simulink model "MATLAB Simulink Model"  (R2020b)
settings: Solver=ode4  StartTime=0.0  StopTime=1  RelTol=1e-3
InitFcn:
  | clear;
  | clc;
  | 
  | %Motor Parameters
  | r1 = 1.405;
  | l1  = 0.005839;
  | r2 = 1.395;
  | l2 = 0.005839;
  | Lm = 0.1722;
  | 
  | %Motor Rated Values
  | Vrat = 400;
  | frat = 50;
  | 
  | x1 = 2*pi*frat*l1;
  | x2 = 2*pi*frat*l2;
  | Xm = 2*pi*frat*Lm;
  | Prat = 4*1000;
  | Nrat = 1430;
  | Ns = 120*frat/4;
  | nrat = Nrat*2*pi/60;
  | ns = Ns*2*pi/60;
  | srat = (Ns-Nrat)/Ns;
  | 
  | E1 = Vrat/sqrt(3); %phase voltage
  | IL = E1/( (r1 + (1i*x1) ) + ( ( (1i*x2) +(r2/srat) )*1i*Xm / ( (1i*Xm) + (1i*x2) + (r2/srat) ) ) );
  | E2 = E1 - (IL*(r1 + (1i*x1) ) );
  | Trat = (3/(ns))*srat*abs(E2)*abs(E2)*r2/((r2*r2) + (srat*srat*x2*x2));
  | %Trat = Prat/nrat;
  | 
  | %System Variables
  | Tsys = (1e-6);
  | Ts = (100e-6);
  | freq = 50;
  | 
  | m=1*freq/50;
  | %m = 1 * (freq/50);
  | Vbus = (400*sqrt(2)*2/sqrt(3)) / (1.15);
  | 
  | Vref = (Vbus*sqrt(3)/2) * m;
  | delay = Ts/Tsys;
  | 
  | % Motor Starting Parameters
  | inc_time = 0.1;
  | 
  | %Motor Loading time
  | load_time = 0.5;
  | 
  | %No. of Hybrid Zones
  | numzones = 3;
  | 
  | %Load ML model Weights
  | 
  | W1R_s1 = readmatrix('Regression Weights\W1_subnet1_tmp_odd_90.xlsx');
  | b1R_s1 = readmatrix('Regression Weights\b1_subnet1_tmp_odd_90.xlsx');
  | W1R_s2 = readmatrix('Regression Weights\W1_subnet2_tmp_odd_90.xlsx');
  | b1R_s2 = readmatrix('Regression Weights\b1_subnet2_tmp_odd_90.xlsx');
  | 
  | W2R = readmatrix('Regression Weights\W2_subnet_tmp_odd_90.xlsx');
  | b2R = readmatrix('Regression Weights\b2_subnet_tmp_odd_90.xlsx');
  | ... (+9 lines)
libraries: powerlib x72, simulink x55, powerlib_meascontrol x15, dspstat3 x11, dspsigops x1
(part 2 of 5)

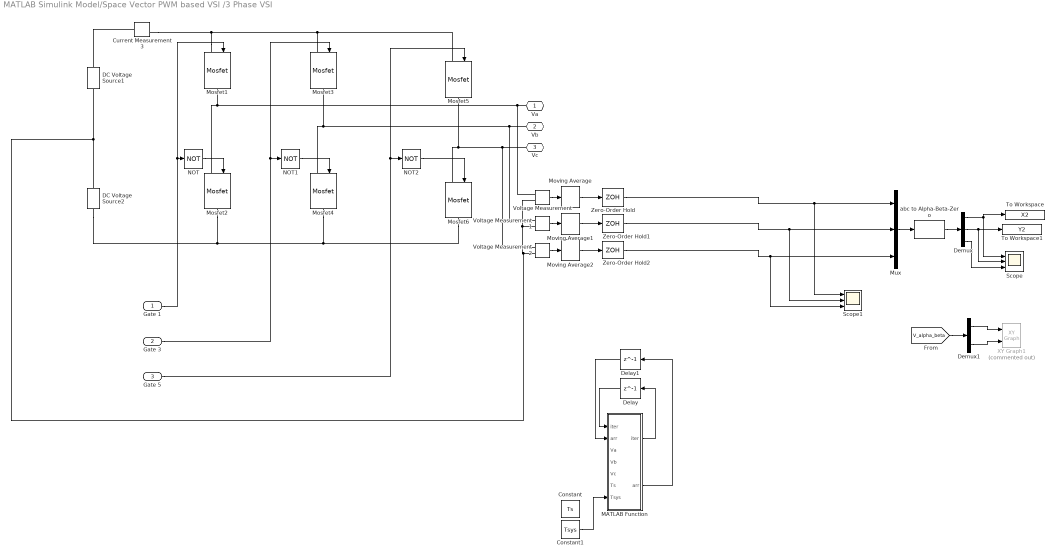
== system MATLAB Simulink Model/Space Vector PWM based VSI /3 Phase VSI ==
  Gate 1 : Inport
  Gate 3 : Inport  Port=2
  Gate 5 : Inport  Port=3
  Constant : Constant  Value=Ts  SampleTime=Tsys
  Constant1 : Constant  Value=Tsys  SampleTime=Tsys
  Current Measurement3 : powerlib/Measurements/Current Measurement  PhasorSimulation=off  OutputType=Complex  PSBequivalent=0
  DC Voltage Source1 : powerlib/Electrical Sources/DC Voltage Source  Amplitude=Vbus/2  Measurements=None
  DC Voltage Source2 : powerlib/Electrical Sources/DC Voltage Source  Amplitude=Vbus/2  Measurements=None
  Delay : Delay  DelayLength=1  SampleTime=Tsys
  Delay1 : Delay  DelayLength=1  SampleTime=Tsys
  Demux : Demux  Outputs=3
  Demux1 : Demux  Outputs=2
  MATLAB Function : MATLAB Function  TreatAsAtomicUnit=on
  Mosfet{1..6} (6 alike) : powerlib/Power Electronics/Mosfet  Ron=1e-6  Lon=0  Rd=1e-6  Vfd=0  IC=0  Rs=1e5  Cs=inf  Measurements=off
  Moving Average : dspstat3/Moving Average  Method=Sliding window  ForgettingFactorPort=off  SpecifyWindowLength=on  WindowLength=int8(Ts/Tsys)  ForgettingFactor=0.9  SimulateUsing=Code generation
  Moving Average1 : dspstat3/Moving Average  Method=Sliding window  ForgettingFactorPort=off  SpecifyWindowLength=on  WindowLength=int8(Ts/Tsys)  ForgettingFactor=0.9  SimulateUsing=Code generation
  Moving Average2 : dspstat3/Moving Average  Method=Sliding window  ForgettingFactorPort=off  SpecifyWindowLength=on  WindowLength=int8(Ts/Tsys)  ForgettingFactor=0.9  SimulateUsing=Code generation
  Mux : Mux  Inputs=3
  NOT : Logic  Operator=NOT  IconShape=distinctive  AllPortsSameDT=off  OutDataTypeStr=boolean
  NOT1 : Logic  Operator=NOT  IconShape=distinctive  AllPortsSameDT=off  OutDataTypeStr=boolean
  NOT2 : Logic  Operator=NOT  IconShape=distinctive  AllPortsSameDT=off  OutDataTypeStr=boolean
  Scope : Scope  NumInputPorts=3
  Scope1 : Scope  NumInputPorts=3
  To Workspace : ToWorkspace  VariableName=X2  SampleTime=-1
  To Workspace1 : ToWorkspace  VariableName=Y2  SampleTime=-1
  Voltage Measurement : powerlib/Measurements/Voltage Measurement  PhasorSimulation=off  OutputType=Complex  PSBequivalent=0
  Voltage Measurement1 : powerlib/Measurements/Voltage Measurement  PhasorSimulation=off  OutputType=Complex  PSBequivalent=0
  Voltage Measurement2 : powerlib/Measurements/Voltage Measurement  PhasorSimulation=off  OutputType=Complex  PSBequivalent=0
  XY Graph1 : simulink/Sinks/XY Graph  Commented=on  xmin=-Vref  xmax=Vref  ymin=-Vref  ymax=Vref  st=Ts
  Zero-Order Hold : ZeroOrderHold  SampleTime=Ts
  Zero-Order Hold1 : ZeroOrderHold  SampleTime=Ts
  Zero-Order Hold2 : ZeroOrderHold  SampleTime=Ts
  abc to Alpha-Beta-Zero : powerlib_meascontrol/Transformations/abc to Alpha-Beta-Zero
  Va : PMIOPort  Side=Right
  Vb : PMIOPort  Port=2  Side=Right
  Vc : PMIOPort  Port=3  Side=Right
  wires:
  Gate 3/1 -> NOT1/1, Mosfet3/1
  NOT1/1 -> Mosfet4/1
  Gate 1/1 -> NOT/1, Mosfet1/1
  Gate 5/1 -> NOT2/1, Mosfet5/1
  NOT/1 -> Mosfet2/1
  NOT2/1 -> Mosfet6/1
  Mux/1 -> abc to Alpha-Beta-Zero/1
  abc to Alpha-Beta-Zero/1 -> Demux/1
  Demux/1 -> To Workspace/1, Scope/1
  Demux/2 -> To Workspace1/1, Scope/2
  Demux/3 -> Scope/3
  [V_alpha_beta] -> Demux1/1
  Demux1/1 -> XY Graph1/1
  Demux1/2 -> XY Graph1/2
  Constant1/1 -> MATLAB Function/7(Tsys)
  MATLAB Function/1(iter) -> Delay/1
  Delay/1 -> MATLAB Function/1("iter ")
  Delay1/1 -> MATLAB Function/2("arr ")
  MATLAB Function/2(arr) -> Delay1/1
  Voltage Measurement/1 -> Moving Average/1
  Voltage Measurement1/1 -> Moving Average1/1
  Voltage Measurement2/1 -> Moving Average2/1
  Moving Average/1 -> Zero-Order Hold/1
  Moving Average1/1 -> Zero-Order Hold1/1
  Moving Average2/1 -> Zero-Order Hold2/1
  Zero-Order Hold/1 -> Scope1/1, Mux/1
  Zero-Order Hold1/1 -> Scope1/2, Mux/2
  Zero-Order Hold2/1 -> Scope1/3, Mux/3
  connections:
  Mosfet6/LConn1 -- Voltage Measurement2/LConn1 -- Vc/RConn1 -- Mosfet5/RConn1
  Mosfet4/LConn1 -- Voltage Measurement1/LConn1 -- Vb/RConn1 -- Mosfet3/RConn1
  Current Measurement3/LConn1 -- DC Voltage Source1/RConn1
  Mosfet1/LConn1 -- Current Measurement3/RConn1 -- Mosfet5/LConn1 -- Mosfet3/LConn1
  Mosfet2/LConn1 -- Voltage Measurement/LConn1 -- Va/RConn1 -- Mosfet1/RConn1
  Mosfet4/RConn1 -- DC Voltage Source2/LConn1 -- Mosfet2/RConn1 -- Mosfet6/RConn1
  DC Voltage Source2/RConn1 -- DC Voltage Source1/LConn1 -- Voltage Measurement1/LConn2 -- Voltage Measurement/LConn2 -- Voltage Measurement2/LConn2

== system MATLAB Simulink Model/Space Vector PWM based VSI /Gate Pulse Generator ==
  S1 : Inport
  S3 : Inport  Port=2
  S5 : Inport  Port=3
  sector : Inport  Port=4
  Constant : Constant  Value=Ts
  Constant1 : Constant  Value=Tsys
  Data Type Conversion : DataTypeConversion  OutDataTypeStr=boolean  RndMeth=Ceiling
  Data Type Conversion1 : DataTypeConversion  OutDataTypeStr=boolean  RndMeth=Ceiling
  Data Type Conversion2 : DataTypeConversion  OutDataTypeStr=boolean  RndMeth=Ceiling
  Delay : Delay  DelayLength=1
  Gate Pulse Values : MATLAB Function  TreatAsAtomicUnit=on
  Scope1 : Scope  NumInputPorts=5
  Gate 1 Pulse : Outport
  Gate 3 Pulse : Outport  Port=2
  Gate 5 Pulse : Outport  Port=3
  wires:
  sector/1 -> Scope1/5
  S1/1 -> Gate Pulse Values/2(S1)
  S3/1 -> Gate Pulse Values/3(S3)
  Gate Pulse Values/1(count) -> Delay/1
  Delay/1 -> Gate Pulse Values/1("count ")
  Gate Pulse Values/2(G1) -> Data Type Conversion/1
  Gate Pulse Values/3(G3) -> Data Type Conversion1/1
  Gate Pulse Values/4(G5) -> Data Type Conversion2/1
  Constant/1 -> Gate Pulse Values/5(Ts)
  Constant1/1 -> Gate Pulse Values/6(Tsys)
  S5/1 -> Gate Pulse Values/4(S5)
  Data Type Conversion/1 -> Gate 1 Pulse/1, Scope1/1
  Data Type Conversion1/1 -> Scope1/2, Gate 3 Pulse/1
  Data Type Conversion2/1 -> Gate 5 Pulse/1, Scope1/3
  [switchseq] -> Scope1/4

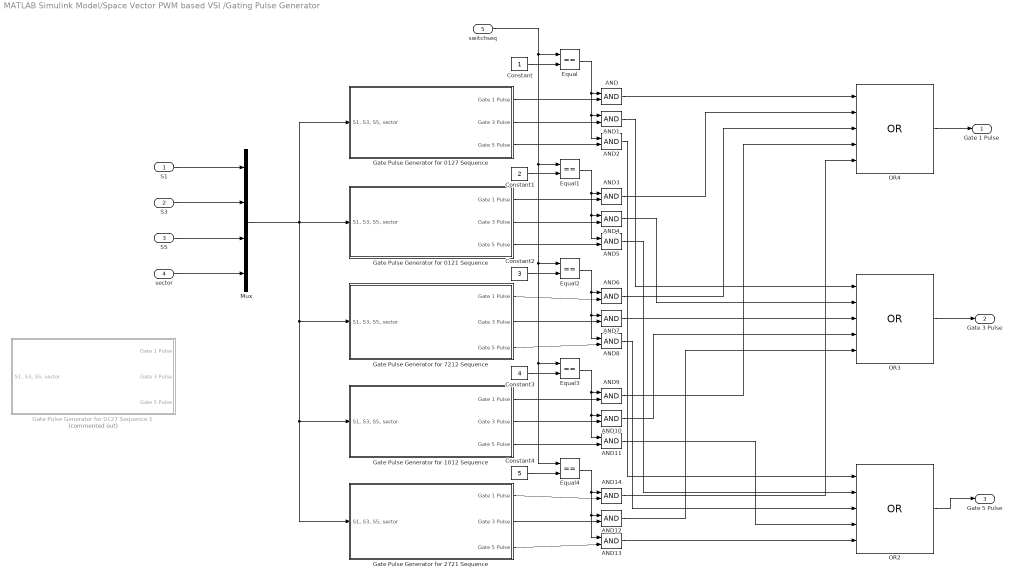
== system MATLAB Simulink Model/Space Vector PWM based VSI /Gating Pulse Generator ==
  S1 : Inport
  S3 : Inport  Port=2
  S5 : Inport  Port=3
  sector : Inport  Port=4
  switchseq : Inport  Port=5
  AND{,1..14} (15 alike) : Logic  IconShape=distinctive  AllPortsSameDT=off  OutDataTypeStr=boolean
  Constant : Constant
  Constant1 : Constant  Value=2
  Constant2 : Constant  Value=3
  Constant3 : Constant  Value=4
  Constant4 : Constant  Value=5
  Equal{,1..4} (5 alike) : RelationalOperator  Operator===  OutDataTypeStr=boolean  RndMeth=Simplest
  Gate Pulse Generator for 0121 Sequence : Subsystem
  Gate Pulse Generator for 0127 Sequence : Subsystem
  Gate Pulse Generator for 0127 Sequence 1 : Subsystem  Commented=on
  Gate Pulse Generator for 1012 Sequence : Subsystem
  Gate Pulse Generator for 2721 Sequence : Subsystem
  Gate Pulse Generator for 7212 Sequence : Subsystem
  Mux : Mux
  OR2 : Logic  Operator=OR  Inputs=5  IconShape=distinctive  AllPortsSameDT=off  OutDataTypeStr=boolean
  OR3 : Logic  Operator=OR  Inputs=5  IconShape=distinctive  AllPortsSameDT=off  OutDataTypeStr=boolean
  OR4 : Logic  Operator=OR  Inputs=5  IconShape=distinctive  AllPortsSameDT=off  OutDataTypeStr=boolean
  Gate 1 Pulse : Outport
  Gate 3 Pulse : Outport  Port=2
  Gate 5 Pulse : Outport  Port=3
  wires:
  sector/1 -> Mux/4
  S5/1 -> Mux/3
  S3/1 -> Mux/2
  S1/1 -> Mux/1
  Mux/1 -> Gate Pulse Generator for 0121 Sequence/1("S1, S3, S5, sector"), Gate Pulse Generator for 0127 Sequence/1("S1, S3, S5, sector"), Gate Pulse Generator for 7212 Sequence/1("S1, S3, S5, sector"), Gate Pulse Generator for 2721 Sequence/1("S1, S3, S5, sector"), Gate Pulse Generator for 1012 Sequence/1("S1, S3, S5, sector")
  Constant/1 -> Equal/2
  Equal/1 -> AND2/1, AND1/1, AND/1
  Gate Pulse Generator for 0121 Sequence/3(Gate 5 Pulse) -> AND5/2
  Gate Pulse Generator for 0121 Sequence/2(Gate 3 Pulse) -> AND4/2
  Equal1/1 -> AND3/1, AND4/1, AND5/1
  Gate Pulse Generator for 0121 Sequence/1(Gate 1 Pulse) -> AND3/2
  Constant1/1 -> Equal1/2
  Constant2/1 -> Equal2/2
  Gate Pulse Generator for 7212 Sequence/1(Gate 1 Pulse) -> AND6/2
  Equal2/1 -> AND8/1, AND7/1, AND6/1
  Gate Pulse Generator for 7212 Sequence/2(Gate 3 Pulse) -> AND7/2
  Gate Pulse Generator for 7212 Sequence/3(Gate 5 Pulse) -> AND8/2
  OR2/1 -> Gate 5 Pulse/1
  OR3/1 -> Gate 3 Pulse/1
  OR4/1 -> Gate 1 Pulse/1
  Gate Pulse Generator for 1012 Sequence/3(Gate 5 Pulse) -> AND11/2
  Gate Pulse Generator for 1012 Sequence/2(Gate 3 Pulse) -> AND10/2
  Equal3/1 -> AND10/1, AND11/1, AND9/1
  Gate Pulse Generator for 1012 Sequence/1(Gate 1 Pulse) -> AND9/2
  Constant3/1 -> Equal3/2
  switchseq/1 -> Equal/1, Equal4/1, Equal3/1, Equal2/1, Equal1/1
  Constant4/1 -> Equal4/2
  Gate Pulse Generator for 2721 Sequence/1(Gate 1 Pulse) -> AND14/2
  Equal4/1 -> AND14/1, AND13/1, AND12/1
  Gate Pulse Generator for 2721 Sequence/2(Gate 3 Pulse) -> AND12/2
  Gate Pulse Generator for 2721 Sequence/3(Gate 5 Pulse) -> AND13/2
  AND/1 -> OR4/1
  AND7/1 -> OR3/3
  AND13/1 -> OR2/5
  AND14/1 -> OR4/5
  AND3/1 -> OR4/2
  AND6/1 -> OR4/3
  AND9/1 -> OR4/4
  AND1/1 -> OR3/1
  AND4/1 -> OR3/2
  AND10/1 -> OR3/4
  AND12/1 -> OR3/5
  AND2/1 -> OR2/1
  AND5/1 -> OR2/2
  AND8/1 -> OR2/3
  AND11/1 -> OR2/4
  Gate Pulse Generator for 0127 Sequence/3(Gate 5 Pulse) -> AND2/2
  Gate Pulse Generator for 0127 Sequence/2(Gate 3 Pulse) -> AND1/2
  Gate Pulse Generator for 0127 Sequence/1(Gate 1 Pulse) -> AND/2

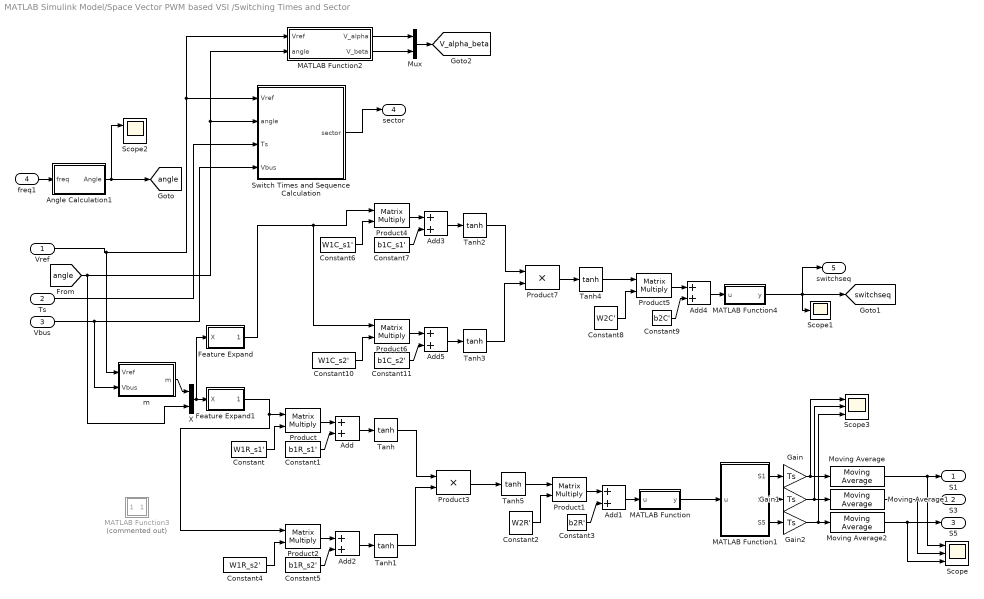
== system MATLAB Simulink Model/Space Vector PWM based VSI /Switching Times and Sector ==
  Vref : Inport
  Ts : Inport  Port=2
  Vbus : Inport  Port=3
  freq1 : Inport  Port=4
  Add{,1..5} (6 alike) : Sum
  Angle Calculation1 : Subsystem
  Constant : Constant  Value=W1R_s1'
  Constant1 : Constant  Value=b1R_s1'
  Constant10 : Constant  Value=W1C_s2'
  Constant11 : Constant  Value=b1C_s2'
  Constant2 : Constant  Value=W2R'
  Constant3 : Constant  Value=b2R'
  Constant4 : Constant  Value=W1R_s2'
  Constant5 : Constant  Value=b1R_s2'
  Constant6 : Constant  Value=W1C_s1'
  Constant7 : Constant  Value=b1C_s1'
  Constant8 : Constant  Value=W2C'
  Constant9 : Constant  Value=b2C'
  Feature Expand : MATLAB Function  TreatAsAtomicUnit=on
  Feature Expand1 : MATLAB Function  TreatAsAtomicUnit=on
  Gain : Gain  Gain=Ts
  Gain1 : Gain  Gain=Ts
  Gain2 : Gain  Gain=Ts
  MATLAB Function : MATLAB Function  TreatAsAtomicUnit=on
  MATLAB Function1 : MATLAB Function  TreatAsAtomicUnit=on
  MATLAB Function2 : MATLAB Function  TreatAsAtomicUnit=on
  MATLAB Function3 : MATLAB Function  Commented=on  TreatAsAtomicUnit=on
  MATLAB Function4 : MATLAB Function  TreatAsAtomicUnit=on
  Moving Average : dspstat3/Moving Average  Method=Sliding window  ForgettingFactorPort=off  SpecifyWindowLength=on  WindowLength=1  ForgettingFactor=0.9  SimulateUsing=Code generation
  Moving Average1 : dspstat3/Moving Average  Method=Sliding window  ForgettingFactorPort=off  SpecifyWindowLength=on  WindowLength=1  ForgettingFactor=0.9  SimulateUsing=Code generation
  Moving Average2 : dspstat3/Moving Average  Method=Sliding window  ForgettingFactorPort=off  SpecifyWindowLength=on  WindowLength=1  ForgettingFactor=0.9  SimulateUsing=Code generation
  Mux : Mux  Inputs=2
  Product{,1..2,4..6} (6 alike) : Product  Multiplication=Matrix(*)
  Product3 : Product
  Product7 : Product
  Scope : Scope  NumInputPorts=3
  Scope1 : Scope
  Scope2 : Scope  NumInputPorts=2
  Scope3 : Scope  NumInputPorts=3
  Switch Times and Sequence Calculation : MATLAB Function  TreatAsAtomicUnit=on
  Tanh{,1..5} (6 alike) : Trigonometry  Operator=tanh
  X : Concatenate
  m : MATLAB Function  TreatAsAtomicUnit=on
  S1 : Outport
  S3 : Outport  Port=2
  S5 : Outport  Port=3
  sector : Outport  Port=4
  switchseq : Outport  Port=5
  tag scope: V_alpha_beta=global, angle=global, switchseq=global
  wires:
  Vref/1 -> m/1(Vref), MATLAB Function2/1(Vref), Switch Times and Sequence Calculation/1(Vref)
  Ts/1 -> Switch Times and Sequence Calculation/3(Ts)
  [angle] -> X/2, MATLAB Function2/2(angle), Switch Times and Sequence Calculation/2(angle)
  Switch Times and Sequence Calculation/1(sector) -> sector/1
  Constant/1 -> Product/2
  Product/1 -> Add/1
  Constant1/1 -> Add/2
  Constant3/1 -> Add1/2
  Product1/1 -> Add1/1
  Constant2/1 -> Product1/2
  Add/1 -> Tanh/1
  Add1/1 -> MATLAB Function/1(u)
  MATLAB Function/1(y) -> MATLAB Function1/1(u)
  X/1 -> Feature Expand/1(X), Feature Expand1/1(X)
  freq1/1 -> Angle Calculation1/1(freq)
  Angle Calculation1/1(Angle) -> Scope2/1, [angle]
  MATLAB Function1/1(S1) -> Gain/1
  MATLAB Function1/3(S5) -> Gain2/1
  MATLAB Function1/2(S3) -> Gain1/1
  m/1(m) -> X/1
  Vbus/1 -> m/2(Vbus), Switch Times and Sequence Calculation/4(Vbus)
  Add2/1 -> Tanh1/1
  Constant5/1 -> Add2/2
  Product2/1 -> Add2/1
  Constant4/1 -> Product2/2
  Tanh1/1 -> Product3/2
  Tanh/1 -> Product3/1
  MATLAB Function2/1(V_alpha) -> Mux/1
  MATLAB Function2/2(V_beta) -> Mux/2
  Mux/1 -> [V_alpha_beta]
  Tanh2/1 -> Product7/1
  Tanh3/1 -> Product7/2
  Constant10/1 -> Product6/2
  Product6/1 -> Add5/1
  Constant11/1 -> Add5/2
  Add5/1 -> Tanh3/1
  Feature Expand/1(new_X) -> Product4/1, Product6/1
  MATLAB Function4/1(y) -> switchseq/1, Scope1/1, [switchseq]
  Add4/1 -> MATLAB Function4/1(u)
  Add3/1 -> Tanh2/1
  Constant8/1 -> Product5/2
  Product5/1 -> Add4/1
  Constant9/1 -> Add4/2
  Constant7/1 -> Add3/2
  Product4/1 -> Add3/1
  Constant6/1 -> Product4/2
  Product7/1 -> Tanh4/1
  Tanh4/1 -> Product5/1
  Tanh5/1 -> Product1/1
  Product3/1 -> Tanh5/1
  Feature Expand1/1(new_X) -> Product/1, Product2/1
  Gain/1 -> Scope3/1, Moving Average/1
  Moving Average/1 -> Scope/1, S1/1
  Gain1/1 -> Scope3/2, Moving Average1/1
  Gain2/1 -> Scope3/3, Moving Average2/1
  Moving Average1/1 -> Scope/2, S3/1
  Moving Average2/1 -> Scope/3, S5/1

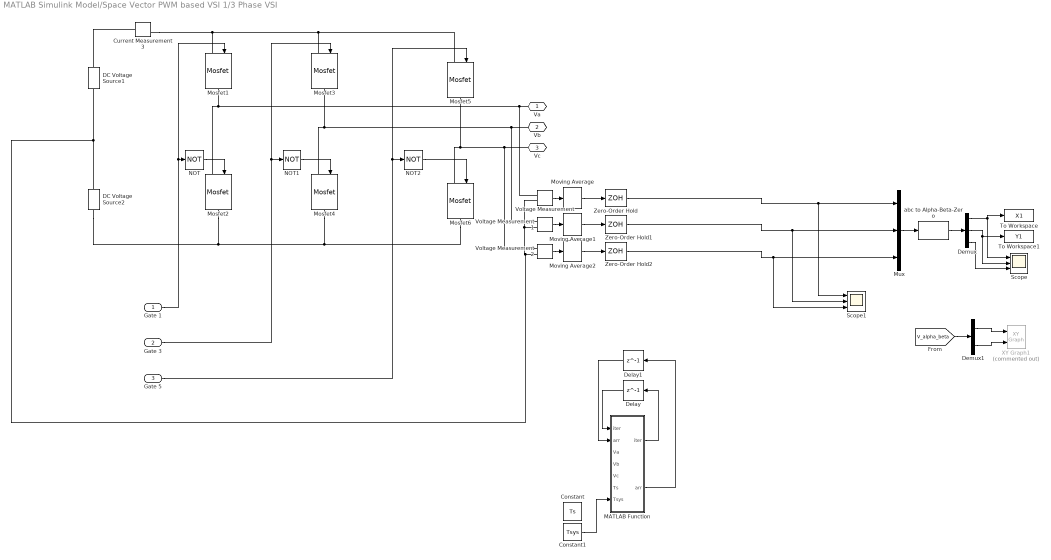
== system MATLAB Simulink Model/Space Vector PWM based VSI 1/3 Phase VSI ==
  Gate 1 : Inport
  Gate 3 : Inport  Port=2
  Gate 5 : Inport  Port=3
  Constant : Constant  Value=Ts  SampleTime=Tsys
  Constant1 : Constant  Value=Tsys  SampleTime=Tsys
  Current Measurement3 : powerlib/Measurements/Current Measurement  PhasorSimulation=off  OutputType=Complex  PSBequivalent=0
  DC Voltage Source1 : powerlib/Electrical Sources/DC Voltage Source  Amplitude=Vbus/2  Measurements=None
  DC Voltage Source2 : powerlib/Electrical Sources/DC Voltage Source  Amplitude=Vbus/2  Measurements=None
  Delay : Delay  DelayLength=1  SampleTime=Tsys
  Delay1 : Delay  DelayLength=1  SampleTime=Tsys
  Demux : Demux  Outputs=3
  Demux1 : Demux  Outputs=2
  MATLAB Function : MATLAB Function  TreatAsAtomicUnit=on
  Mosfet{1..6} (6 alike) : powerlib/Power Electronics/Mosfet  Ron=1e-6  Lon=0  Rd=1e-6  Vfd=0  IC=0  Rs=1e5  Cs=inf  Measurements=off
  Moving Average : dspstat3/Moving Average  Method=Sliding window  ForgettingFactorPort=off  SpecifyWindowLength=on  WindowLength=int8(Ts/Tsys)  ForgettingFactor=0.9  SimulateUsing=Code generation
  Moving Average1 : dspstat3/Moving Average  Method=Sliding window  ForgettingFactorPort=off  SpecifyWindowLength=on  WindowLength=int8(Ts/Tsys)  ForgettingFactor=0.9  SimulateUsing=Code generation
  Moving Average2 : dspstat3/Moving Average  Method=Sliding window  ForgettingFactorPort=off  SpecifyWindowLength=on  WindowLength=int8(Ts/Tsys)  ForgettingFactor=0.9  SimulateUsing=Code generation
  Mux : Mux  Inputs=3
  NOT : Logic  Operator=NOT  IconShape=distinctive  AllPortsSameDT=off  OutDataTypeStr=boolean
  NOT1 : Logic  Operator=NOT  IconShape=distinctive  AllPortsSameDT=off  OutDataTypeStr=boolean
  NOT2 : Logic  Operator=NOT  IconShape=distinctive  AllPortsSameDT=off  OutDataTypeStr=boolean
  Scope : Scope  NumInputPorts=3
  Scope1 : Scope  NumInputPorts=3
  To Workspace : ToWorkspace  VariableName=X1  SampleTime=-1
  To Workspace1 : ToWorkspace  VariableName=Y1  SampleTime=-1
  Voltage Measurement : powerlib/Measurements/Voltage Measurement  PhasorSimulation=off  OutputType=Complex  PSBequivalent=0
  Voltage Measurement1 : powerlib/Measurements/Voltage Measurement  PhasorSimulation=off  OutputType=Complex  PSBequivalent=0
  Voltage Measurement2 : powerlib/Measurements/Voltage Measurement  PhasorSimulation=off  OutputType=Complex  PSBequivalent=0
  XY Graph1 : simulink/Sinks/XY Graph  Commented=on  xmin=-Vref  xmax=Vref  ymin=-Vref  ymax=Vref  st=Ts
  Zero-Order Hold : ZeroOrderHold  SampleTime=Ts
  Zero-Order Hold1 : ZeroOrderHold  SampleTime=Ts
  Zero-Order Hold2 : ZeroOrderHold  SampleTime=Ts
  abc to Alpha-Beta-Zero : powerlib_meascontrol/Transformations/abc to Alpha-Beta-Zero
  Va : PMIOPort  Side=Right
  Vb : PMIOPort  Port=2  Side=Right
  Vc : PMIOPort  Port=3  Side=Right
  wires:
  Zero-Order Hold2/1 -> Mux/3, Scope1/3
  Zero-Order Hold1/1 -> Mux/2, Scope1/2
  Zero-Order Hold/1 -> Mux/1, Scope1/1
  Moving Average2/1 -> Zero-Order Hold2/1
  Moving Average1/1 -> Zero-Order Hold1/1
  Moving Average/1 -> Zero-Order Hold/1
  Voltage Measurement2/1 -> Moving Average2/1
  Voltage Measurement1/1 -> Moving Average1/1
  Voltage Measurement/1 -> Moving Average/1
  MATLAB Function/2(arr) -> Delay1/1
  Delay1/1 -> MATLAB Function/2("arr ")
  Delay/1 -> MATLAB Function/1("iter ")
  MATLAB Function/1(iter) -> Delay/1
  Constant1/1 -> MATLAB Function/7(Tsys)
  Demux1/2 -> XY Graph1/2
  Demux1/1 -> XY Graph1/1
  [V_alpha_beta] -> Demux1/1
  Demux/3 -> Scope/3
  Demux/2 -> To Workspace1/1, Scope/2
  Demux/1 -> To Workspace/1, Scope/1
  abc to Alpha-Beta-Zero/1 -> Demux/1
  Mux/1 -> abc to Alpha-Beta-Zero/1
  NOT2/1 -> Mosfet6/1
  NOT/1 -> Mosfet2/1
  Gate 5/1 -> Mosfet5/1, NOT2/1
  Gate 1/1 -> Mosfet1/1, NOT/1
  NOT1/1 -> Mosfet4/1
  Gate 3/1 -> Mosfet3/1, NOT1/1
  connections:
  Voltage Measurement2/LConn2 -- Voltage Measurement/LConn2 -- Voltage Measurement1/LConn2 -- DC Voltage Source1/LConn1 -- DC Voltage Source2/RConn1
  Mosfet6/RConn1 -- Mosfet2/RConn1 -- DC Voltage Source2/LConn1 -- Mosfet4/RConn1
  Mosfet1/RConn1 -- Va/RConn1 -- Voltage Measurement/LConn1 -- Mosfet2/LConn1
  Mosfet3/LConn1 -- Mosfet5/LConn1 -- Current Measurement3/RConn1 -- Mosfet1/LConn1
  Current Measurement3/LConn1 -- DC Voltage Source1/RConn1
  Mosfet3/RConn1 -- Vb/RConn1 -- Voltage Measurement1/LConn1 -- Mosfet4/LConn1
  Mosfet5/RConn1 -- Vc/RConn1 -- Voltage Measurement2/LConn1 -- Mosfet6/LConn1

== system MATLAB Simulink Model/Space Vector PWM based VSI 1/Gate Pulse Generator ==
  S1 : Inport
  S3 : Inport  Port=2
  S5 : Inport  Port=3
  sector : Inport  Port=4
  Constant : Constant  Value=Ts
  Constant1 : Constant  Value=Tsys
  Data Type Conversion : DataTypeConversion  OutDataTypeStr=boolean  RndMeth=Ceiling
  Data Type Conversion1 : DataTypeConversion  OutDataTypeStr=boolean  RndMeth=Ceiling
  Data Type Conversion2 : DataTypeConversion  OutDataTypeStr=boolean  RndMeth=Ceiling
  Delay : Delay  DelayLength=1
  Gate Pulse Values : MATLAB Function  TreatAsAtomicUnit=on
  Scope1 : Scope  NumInputPorts=5
  Gate 1 Pulse : Outport
  Gate 3 Pulse : Outport  Port=2
  Gate 5 Pulse : Outport  Port=3
  wires:
  [switchseq] -> Scope1/4
  Data Type Conversion2/1 -> Scope1/3, Gate 5 Pulse/1
  Data Type Conversion1/1 -> Gate 3 Pulse/1, Scope1/2
  Data Type Conversion/1 -> Scope1/1, Gate 1 Pulse/1
  S5/1 -> Gate Pulse Values/4(S5)
  Constant1/1 -> Gate Pulse Values/6(Tsys)
  Constant/1 -> Gate Pulse Values/5(Ts)
  Gate Pulse Values/4(G5) -> Data Type Conversion2/1
  Gate Pulse Values/3(G3) -> Data Type Conversion1/1
  Gate Pulse Values/2(G1) -> Data Type Conversion/1
  Delay/1 -> Gate Pulse Values/1("count ")
  Gate Pulse Values/1(count) -> Delay/1
  S3/1 -> Gate Pulse Values/3(S3)
  S1/1 -> Gate Pulse Values/2(S1)
  sector/1 -> Scope1/5

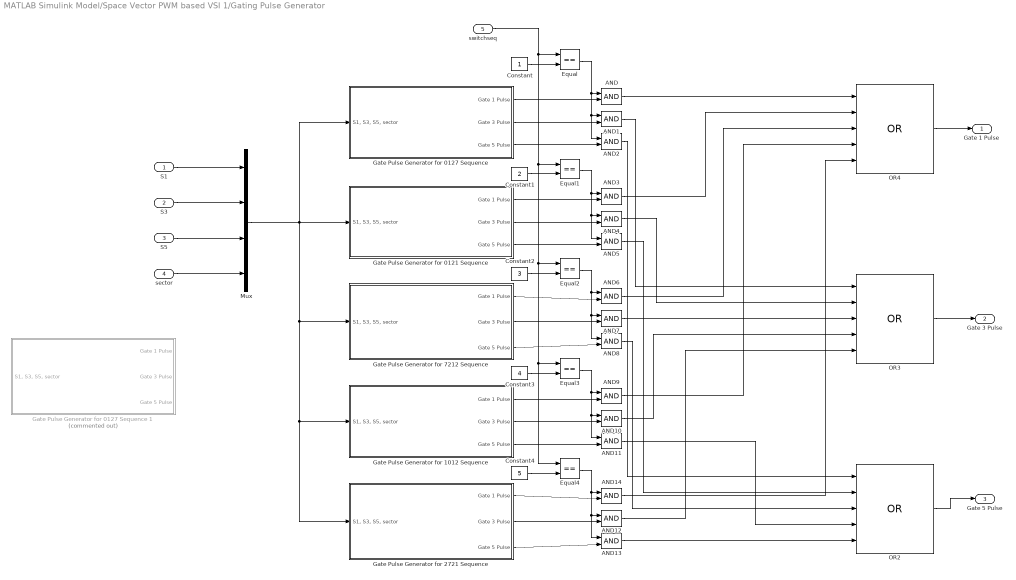
== system MATLAB Simulink Model/Space Vector PWM based VSI 1/Gating Pulse Generator ==
  S1 : Inport
  S3 : Inport  Port=2
  S5 : Inport  Port=3
  sector : Inport  Port=4
  switchseq : Inport  Port=5
  AND{,1..14} (15 alike) : Logic  IconShape=distinctive  AllPortsSameDT=off  OutDataTypeStr=boolean
  Constant : Constant
  Constant1 : Constant  Value=2
  Constant2 : Constant  Value=3
  Constant3 : Constant  Value=4
  Constant4 : Constant  Value=5
  Equal{,1..4} (5 alike) : RelationalOperator  Operator===  OutDataTypeStr=boolean  RndMeth=Simplest
  Gate Pulse Generator for 0121 Sequence : Subsystem
  Gate Pulse Generator for 0127 Sequence : Subsystem
  Gate Pulse Generator for 0127 Sequence 1 : Subsystem  Commented=on
  Gate Pulse Generator for 1012 Sequence : Subsystem
  Gate Pulse Generator for 2721 Sequence : Subsystem
  Gate Pulse Generator for 7212 Sequence : Subsystem
  Mux : Mux
  OR2 : Logic  Operator=OR  Inputs=5  IconShape=distinctive  AllPortsSameDT=off  OutDataTypeStr=boolean
  OR3 : Logic  Operator=OR  Inputs=5  IconShape=distinctive  AllPortsSameDT=off  OutDataTypeStr=boolean
  OR4 : Logic  Operator=OR  Inputs=5  IconShape=distinctive  AllPortsSameDT=off  OutDataTypeStr=boolean
  Gate 1 Pulse : Outport
  Gate 3 Pulse : Outport  Port=2
  Gate 5 Pulse : Outport  Port=3
  wires:
  Gate Pulse Generator for 0127 Sequence/1(Gate 1 Pulse) -> AND/2
  Gate Pulse Generator for 0127 Sequence/2(Gate 3 Pulse) -> AND1/2
  Gate Pulse Generator for 0127 Sequence/3(Gate 5 Pulse) -> AND2/2
  AND11/1 -> OR2/4
  AND8/1 -> OR2/3
  AND5/1 -> OR2/2
  AND2/1 -> OR2/1
  AND12/1 -> OR3/5
  AND10/1 -> OR3/4
  AND4/1 -> OR3/2
  AND1/1 -> OR3/1
  AND9/1 -> OR4/4
  AND6/1 -> OR4/3
  AND3/1 -> OR4/2
  AND14/1 -> OR4/5
  AND13/1 -> OR2/5
  AND7/1 -> OR3/3
  AND/1 -> OR4/1
  Gate Pulse Generator for 2721 Sequence/3(Gate 5 Pulse) -> AND13/2
  Gate Pulse Generator for 2721 Sequence/2(Gate 3 Pulse) -> AND12/2
  Equal4/1 -> AND12/1, AND13/1, AND14/1
  Gate Pulse Generator for 2721 Sequence/1(Gate 1 Pulse) -> AND14/2
  Constant4/1 -> Equal4/2
  switchseq/1 -> Equal1/1, Equal2/1, Equal3/1, Equal4/1, Equal/1
  Constant3/1 -> Equal3/2
  Gate Pulse Generator for 1012 Sequence/1(Gate 1 Pulse) -> AND9/2
  Equal3/1 -> AND9/1, AND11/1, AND10/1
  Gate Pulse Generator for 1012 Sequence/2(Gate 3 Pulse) -> AND10/2
  Gate Pulse Generator for 1012 Sequence/3(Gate 5 Pulse) -> AND11/2
  OR4/1 -> Gate 1 Pulse/1
  OR3/1 -> Gate 3 Pulse/1
  OR2/1 -> Gate 5 Pulse/1
  Gate Pulse Generator for 7212 Sequence/3(Gate 5 Pulse) -> AND8/2
  Gate Pulse Generator for 7212 Sequence/2(Gate 3 Pulse) -> AND7/2
  Equal2/1 -> AND6/1, AND7/1, AND8/1
  Gate Pulse Generator for 7212 Sequence/1(Gate 1 Pulse) -> AND6/2
  Constant2/1 -> Equal2/2
  Constant1/1 -> Equal1/2
  Gate Pulse Generator for 0121 Sequence/1(Gate 1 Pulse) -> AND3/2
  Equal1/1 -> AND5/1, AND4/1, AND3/1
  Gate Pulse Generator for 0121 Sequence/2(Gate 3 Pulse) -> AND4/2
  Gate Pulse Generator for 0121 Sequence/3(Gate 5 Pulse) -> AND5/2
  Equal/1 -> AND/1, AND1/1, AND2/1
  Constant/1 -> Equal/2
  Mux/1 -> Gate Pulse Generator for 1012 Sequence/1("S1, S3, S5, sector"), Gate Pulse Generator for 2721 Sequence/1("S1, S3, S5, sector"), Gate Pulse Generator for 7212 Sequence/1("S1, S3, S5, sector"), Gate Pulse Generator for 0127 Sequence/1("S1, S3, S5, sector"), Gate Pulse Generator for 0121 Sequence/1("S1, S3, S5, sector")
  S1/1 -> Mux/1
  S3/1 -> Mux/2
  S5/1 -> Mux/3
  sector/1 -> Mux/4

== system MATLAB Simulink Model/Space Vector PWM based VSI 1/Switching Times and Sector ==
  Vref : Inport
  Ts : Inport  Port=2
  Vbus : Inport  Port=3
  freq1 : Inport  Port=4
  Angle Calculation1 : Subsystem
  Scope : Scope  NumInputPorts=3
  Scope2 : Scope  NumInputPorts=2
  Switch Times and Sequence Calculation : MATLAB Function  TreatAsAtomicUnit=on
  S1 : Outport
  S3 : Outport  Port=2
  S5 : Outport  Port=3
  sector : Outport  Port=4
  switchseq : Outport  Port=5
  wires:
  ? -> ?
  Vbus/1 -> Switch Times and Sequence Calculation/4(Vbus)
  Angle Calculation1/1(Angle) -> Scope2/1
  freq1/1 -> Angle Calculation1/1(freq)
  Switch Times and Sequence Calculation/4(sector) -> sector/1
  [angle] -> Switch Times and Sequence Calculation/2(angle)
  Ts/1 -> Switch Times and Sequence Calculation/3(Ts)
  Vref/1 -> Switch Times and Sequence Calculation/1(Vref)
  Switch Times and Sequence Calculation/3(S5) -> Scope/3, S5/1
  Switch Times and Sequence Calculation/2(S3) -> Scope/2, S3/1
  Switch Times and Sequence Calculation/1(S1) -> Scope/1, S1/1
  Switch Times and Sequence Calculation/5(swseq) -> switchseq/1

== system MATLAB Simulink Model/15 Hz System/Space Vector PWM based VSI 1/3 Phase VSI ==
  Gate 1 : Inport
  Gate 3 : Inport  Port=2
  Gate 5 : Inport  Port=3
  Current Measurement3 : powerlib/Measurements/Current Measurement  PhasorSimulation=off  OutputType=Complex  PSBequivalent=0
  DC Voltage Source1 : powerlib/Electrical Sources/DC Voltage Source  Amplitude=Vbus  Measurements=None
  Mosfet{1..6} (6 alike) : powerlib/Power Electronics/Mosfet  Ron=1e-6  Lon=0  Rd=1e-6  Vfd=0  IC=0  Rs=1e5  Cs=inf  Measurements=on
  NOT : Logic  Operator=NOT  IconShape=distinctive  AllPortsSameDT=off  OutDataTypeStr=boolean
  NOT1 : Logic  Operator=NOT  IconShape=distinctive  AllPortsSameDT=off  OutDataTypeStr=boolean
  NOT2 : Logic  Operator=NOT  IconShape=distinctive  AllPortsSameDT=off  OutDataTypeStr=boolean
  Va : PMIOPort  Side=Right
  Vb : PMIOPort  Port=2  Side=Right
  Vc : PMIOPort  Port=3  Side=Right
  wires:
  Gate 3/1 -> NOT1/1, Mosfet3/1
  NOT1/1 -> Mosfet4/1
  Gate 1/1 -> NOT/1, Mosfet1/1
  Gate 5/1 -> NOT2/1, Mosfet5/1
  NOT/1 -> Mosfet2/1
  NOT2/1 -> Mosfet6/1
  connections:
  Mosfet6/LConn1 -- Vc/RConn1 -- Mosfet5/RConn1
  Mosfet4/LConn1 -- Vb/RConn1 -- Mosfet3/RConn1
  Current Measurement3/LConn1 -- DC Voltage Source1/RConn1
  Mosfet1/LConn1 -- Current Measurement3/RConn1 -- Mosfet5/LConn1 -- Mosfet3/LConn1
  Mosfet2/LConn1 -- Va/RConn1 -- Mosfet1/RConn1
  Mosfet4/RConn1 -- DC Voltage Source1/LConn1 -- Mosfet2/RConn1 -- Mosfet6/RConn1

== system MATLAB Simulink Model/15 Hz System/Space Vector PWM based VSI 1/Gate Pulse Generator ==
  "S1, S3, S5, sector" : Inport
  Carrier : simulink/Sources/Repeating Sequence  rep_seq_t=[0 Ts/2 Ts]  rep_seq_y=[Ts 0 Ts]
  Demux : Demux
  G1 : RelationalOperator  OutDataTypeStr=boolean  RndMeth=Simplest
  G3 : RelationalOperator  OutDataTypeStr=boolean  RndMeth=Simplest
  G5 : RelationalOperator  OutDataTypeStr=boolean  RndMeth=Simplest
  Scope : Scope  NumInputPorts=4
  Gate 1 Pulse : Outport
  Gate 3 Pulse : Outport  Port=2
  Gate 5 Pulse : Outport  Port=3
  tag scope: sector1=global
  wires:
  "S1, S3, S5, sector"/1 -> Demux/1
  Demux/4 -> [sector1], Scope/4
  Demux/2 -> G3/1
  Demux/1 -> G1/1
  Carrier/1 -> G5/2, G3/2, G1/2
  G1/1 -> Scope/1, Gate 1 Pulse/1
  Demux/3 -> G5/1
  G3/1 -> Scope/2, Gate 3 Pulse/1
  G5/1 -> Scope/3, Gate 5 Pulse/1

== system MATLAB Simulink Model/15 Hz System/Space Vector PWM based VSI 1/Switching Times and Sector ==
  Vref : Inport
  Ts : Inport  Port=2
  Vbus : Inport  Port=3
  Angle to Sector and Theta : Subsystem
  Mux3 : Mux
  PLL : powerlib_meascontrol/PLL/PLL  Fmin=45  Par_Init=[0, 50]  ParK=[180, 3200, 1]  TcD=1e-4  MaxRateChangeFreq=12  FilterCutOffFreq=25  Ts=0  AGC=on
      settings: SourceProductBaseCode=PS
  Scope : Scope
  Scope2 : Scope  NumInputPorts=2
  Scope3 : Scope  NumInputPorts=3
  Switching times of all switches : MATLAB Function  TreatAsAtomicUnit=on
  Vas : Sin  Frequency=2*pi*15  SampleTime=0
  "S1, S3, S5, sector" : Outport
  tag scope: wt1=global
  wires:
  Angle to Sector and Theta/1(Sector) -> Mux3/4, Switching times of all switches/4(sector)
  Angle to Sector and Theta/2(theta) -> Scope2/2, Switching times of all switches/2(theta)
  Switching times of all switches/2(S3) -> Scope3/2, Mux3/2
  Switching times of all switches/3(S5) -> Scope3/3, Mux3/3
  Ts/1 -> Switching times of all switches/3(Ts)
  PLL/2 -> [wt1], Angle to Sector and Theta/1(angle), Scope2/1
  Vas/1 -> PLL/1
  Switching times of all switches/1(S1) -> Scope3/1, Mux3/1
  PLL/1 -> Scope/1
  Mux3/1 -> "S1, S3, S5, sector"/1
  Vref/1 -> Switching times of all switches/1(Vref)
  Vbus/1 -> Switching times of all switches/5(Vbus)

== system MATLAB Simulink Model/Space Vector PWM based VSI /Gating Pulse Generator/Gate Pulse Generator for 0121 Sequence ==
  "S1, S3, S5, sector" : Inport
  AND{,1..5} (6 alike) : Logic  IconShape=distinctive  AllPortsSameDT=off  OutDataTypeStr=boolean
  Constant : Constant  Value=2
  Data Type Conversion : DataTypeConversion
  Demux : Demux
  For Even Sector : Subsystem
  For Odd Sector : Subsystem
  Mod : Math  Operator=mod  SaturateOnIntegerOverflow=on
  Mux : Mux  Inputs=3
  NOT : Logic  Operator=NOT  IconShape=distinctive  AllPortsSameDT=off  OutDataTypeStr=boolean
  OR : Logic  Operator=OR  IconShape=distinctive  AllPortsSameDT=off  OutDataTypeStr=boolean
  OR1 : Logic  Operator=OR  IconShape=distinctive  AllPortsSameDT=off  OutDataTypeStr=boolean
  OR2 : Logic  Operator=OR  IconShape=distinctive  AllPortsSameDT=off  OutDataTypeStr=boolean
  Scope1 : Scope  NumInputPorts=4
  Gate 1 Pulse : Outport
  Gate 3 Pulse : Outport  Port=2
  Gate 5 Pulse : Outport  Port=3
  wires:
  For Odd Sector/3(Gate 5 Pulse) -> AND5/1
  OR2/1 -> Scope1/3, Gate 5 Pulse/1
  OR1/1 -> Scope1/2, Gate 3 Pulse/1
  Demux/3 -> Mux/3
  AND4/1 -> OR1/1
  OR/1 -> Scope1/1, Gate 1 Pulse/1
  For Odd Sector/1(Gate 1 Pulse) -> AND3/1
  AND5/1 -> OR2/1
  Demux/2 -> Mux/2
  AND1/1 -> OR1/2
  AND/1 -> OR/2
  Demux/4 -> Scope1/4, Mod/1
  For Even Sector/3(Gate 5 Pulse) -> AND2/1
  For Odd Sector/2(Gate 3 Pulse) -> AND4/1
  For Even Sector/1(Gate 1 Pulse) -> AND/1
  Data Type Conversion/1 -> AND3/2, AND4/2, AND5/2, NOT/1
  AND2/1 -> OR2/2
  Demux/1 -> Mux/1
  Mux/1 -> For Even Sector/1("S1, S3, S5"), For Odd Sector/1("S1, S3, S5")
  For Even Sector/2(Gate 3 Pulse) -> AND1/1
  Constant/1 -> Mod/2
  NOT/1 -> AND/2, AND1/2, AND2/2
  Mod/1 -> Data Type Conversion/1
  "S1, S3, S5, sector"/1 -> Demux/1
  AND3/1 -> OR/1

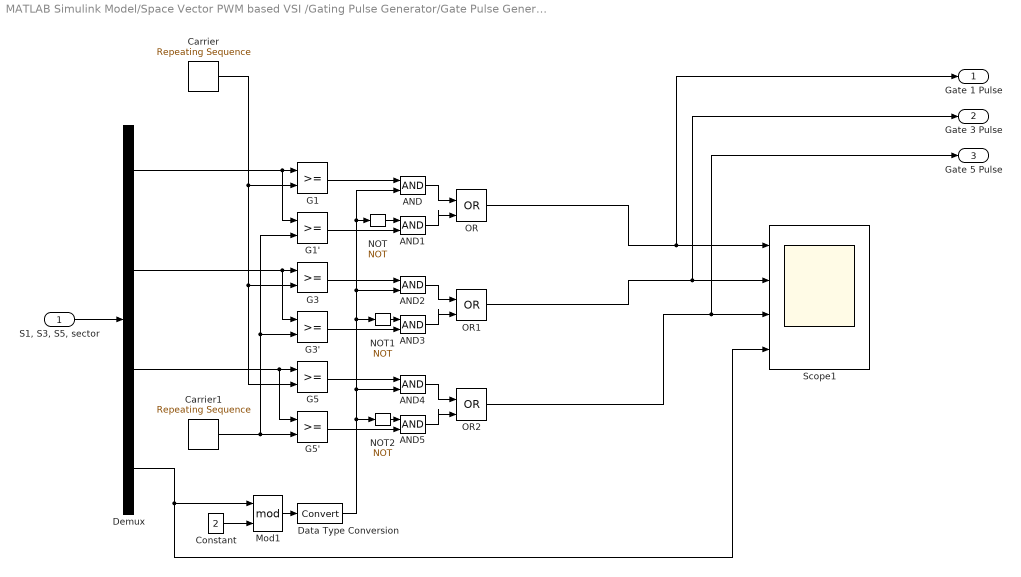
== system MATLAB Simulink Model/Space Vector PWM based VSI /Gating Pulse Generator/Gate Pulse Generator for 0127 Sequence ==
  "S1, S3, S5, sector" : Inport
  AND{,1..5} (6 alike) : Logic  IconShape=distinctive  AllPortsSameDT=off  OutDataTypeStr=boolean
  Carrier : simulink/Sources/Repeating Sequence  rep_seq_t=[0 Ts/2 Ts]  rep_seq_y=[Ts-(1e-16) 0 Ts-(1e-16)]
  Carrier1 : simulink/Sources/Repeating Sequence  rep_seq_t=[0 Ts/2 Ts]  rep_seq_y=[0 Ts-(1e-16) 0]
  Constant : Constant  Value=2
  Data Type Conversion : DataTypeConversion
  Demux : Demux
  G1 : RelationalOperator  OutDataTypeStr=boolean  RndMeth=Simplest
  G1' : RelationalOperator  OutDataTypeStr=boolean  RndMeth=Simplest
  G3 : RelationalOperator  OutDataTypeStr=boolean  RndMeth=Simplest
  G3' : RelationalOperator  OutDataTypeStr=boolean  RndMeth=Simplest
  G5 : RelationalOperator  OutDataTypeStr=boolean  RndMeth=Simplest
  G5' : RelationalOperator  OutDataTypeStr=boolean  RndMeth=Simplest
  Mod1 : Math  Operator=mod  SaturateOnIntegerOverflow=on
  NOT : Logic  Operator=NOT  IconShape=distinctive  AllPortsSameDT=off  OutDataTypeStr=boolean
  NOT1 : Logic  Operator=NOT  IconShape=distinctive  AllPortsSameDT=off  OutDataTypeStr=boolean
  NOT2 : Logic  Operator=NOT  IconShape=distinctive  AllPortsSameDT=off  OutDataTypeStr=boolean
  OR : Logic  Operator=OR  IconShape=distinctive  AllPortsSameDT=off  OutDataTypeStr=boolean
  OR1 : Logic  Operator=OR  IconShape=distinctive  AllPortsSameDT=off  OutDataTypeStr=boolean
  OR2 : Logic  Operator=OR  IconShape=distinctive  AllPortsSameDT=off  OutDataTypeStr=boolean
  Scope1 : Scope  NumInputPorts=4
  Gate 1 Pulse : Outport
  Gate 3 Pulse : Outport  Port=2
  Gate 5 Pulse : Outport  Port=3
  wires:
  G3/1 -> AND2/1
  OR2/1 -> Gate 5 Pulse/1, Scope1/3
  G3'/1 -> AND3/2
  OR/1 -> Gate 1 Pulse/1, Scope1/1
  Constant/1 -> Mod1/2
  AND1/1 -> OR/2
  Data Type Conversion/1 -> NOT2/1, AND4/2, NOT1/1, AND2/2, NOT/1, AND/2
  G5'/1 -> AND5/2
  G5/1 -> AND4/1
  AND5/1 -> OR2/2
  AND4/1 -> OR2/1
  AND/1 -> OR/1
  OR1/1 -> Scope1/2, Gate 3 Pulse/1
  NOT/1 -> AND1/1
  Mod1/1 -> Data Type Conversion/1
  AND3/1 -> OR1/2
  NOT2/1 -> AND5/1
  NOT1/1 -> AND3/1
  Carrier1/1 -> G1'/2, G3'/2, G5'/2
  Demux/1 -> G1'/1, G1/1
  G1'/1 -> AND1/2
  G1/1 -> AND/1
  Carrier/1 -> G5/2, G3/2, G1/2
  AND2/1 -> OR1/1
  "S1, S3, S5, sector"/1 -> Demux/1
  Demux/4 -> Scope1/4, Mod1/1
  Demux/2 -> G3'/1, G3/1
  Demux/3 -> G5'/1, G5/1

== system MATLAB Simulink Model/Space Vector PWM based VSI /Gating Pulse Generator/Gate Pulse Generator for 0127 Sequence 1 ==
  "S1, S3, S5, sector" : Inport
  AND{,1..5} (6 alike) : Logic  IconShape=distinctive  AllPortsSameDT=off  OutDataTypeStr=boolean
  Constant : Constant  Value=2
  Data Type Conversion : DataTypeConversion
  Demux : Demux
  For Even Sector : Subsystem
  For Odd Sector : Subsystem
  Mod : Math  Operator=mod  SaturateOnIntegerOverflow=on
  Mux : Mux  Inputs=3
  NOT : Logic  Operator=NOT  IconShape=distinctive  AllPortsSameDT=off  OutDataTypeStr=boolean
  OR : Logic  Operator=OR  IconShape=distinctive  AllPortsSameDT=off  OutDataTypeStr=boolean
  OR1 : Logic  Operator=OR  IconShape=distinctive  AllPortsSameDT=off  OutDataTypeStr=boolean
  OR2 : Logic  Operator=OR  IconShape=distinctive  AllPortsSameDT=off  OutDataTypeStr=boolean
  Scope1 : Scope  NumInputPorts=4
  Gate 1 Pulse : Outport
  Gate 3 Pulse : Outport  Port=2
  Gate 5 Pulse : Outport  Port=3
  wires:
  "S1, S3, S5, sector"/1 -> Demux/1
  Demux/1 -> Mux/1
  Demux/2 -> Mux/2
  Demux/3 -> Mux/3
  Mux/1 -> For Even Sector/1("S1, S3, S5"), For Odd Sector/1("S1, S3, S1")
  Demux/4 -> Scope1/4, Mod/1
  Constant/1 -> Mod/2
  Mod/1 -> Data Type Conversion/1
  NOT/1 -> AND/2, AND1/2, AND2/2
  For Odd Sector/1(Gate 1 Pulse1) -> AND3/1
  Data Type Conversion/1 -> AND3/2, AND4/2, AND5/2, NOT/1
  AND3/1 -> OR/1
  AND/1 -> OR/2
  AND4/1 -> OR1/1
  AND1/1 -> OR1/2
  AND5/1 -> OR2/1
  AND2/1 -> OR2/2
  OR1/1 -> Scope1/2, Gate 3 Pulse/1
  OR/1 -> Scope1/1, Gate 1 Pulse/1
  OR2/1 -> Scope1/3, Gate 5 Pulse/1
  For Even Sector/1(Gate 1 Pulse) -> AND/1
  For Even Sector/2(Gate 3 Pulse) -> AND1/1
  For Even Sector/3(Gate 5 Pulse) -> AND2/1
  For Odd Sector/2(Gate 3 Pulse1) -> AND4/1
  For Odd Sector/3(Gate 5 Pulse1) -> AND5/1

== system MATLAB Simulink Model/Space Vector PWM based VSI /Gating Pulse Generator/Gate Pulse Generator for 1012 Sequence ==
  "S1, S3, S5, sector" : Inport
  AND{,1..5} (6 alike) : Logic  IconShape=distinctive  AllPortsSameDT=off  OutDataTypeStr=boolean
  Constant : Constant  Value=2
  Data Type Conversion : DataTypeConversion
  Demux : Demux
  For Even Sector : Subsystem
  For Odd Sector : Subsystem
  Mod : Math  Operator=mod  SaturateOnIntegerOverflow=on
  Mux : Mux  Inputs=3
  NOT : Logic  Operator=NOT  IconShape=distinctive  AllPortsSameDT=off  OutDataTypeStr=boolean
  OR : Logic  Operator=OR  IconShape=distinctive  AllPortsSameDT=off  OutDataTypeStr=boolean
  OR1 : Logic  Operator=OR  IconShape=distinctive  AllPortsSameDT=off  OutDataTypeStr=boolean
  OR2 : Logic  Operator=OR  IconShape=distinctive  AllPortsSameDT=off  OutDataTypeStr=boolean
  Scope1 : Scope  NumInputPorts=4
  Gate 1 Pulse : Outport
  Gate 3 Pulse : Outport  Port=2
  Gate 5 Pulse : Outport  Port=3
  wires:
  For Odd Sector/3(Gate 5 Pulse) -> AND5/1
  For Odd Sector/1(Gate 1 Pulse) -> AND3/1
  For Even Sector/3(Gate 5 Pulse) -> AND2/1
  For Even Sector/2(Gate 3 Pulse) -> AND1/1
  OR2/1 -> Scope1/3, Gate 5 Pulse/1
  OR1/1 -> Scope1/2, Gate 3 Pulse/1
  Demux/3 -> Mux/3
  For Even Sector/1(Gate 1 Pulse) -> AND/1
  AND4/1 -> OR1/1
  OR/1 -> Scope1/1, Gate 1 Pulse/1
  AND5/1 -> OR2/1
  Demux/2 -> Mux/2
  AND1/1 -> OR1/2
  AND/1 -> OR/2
  Mod/1 -> Data Type Conversion/1
  Demux/4 -> Scope1/4, Mod/1
  Data Type Conversion/1 -> AND3/2, AND4/2, AND5/2, NOT/1
  AND2/1 -> OR2/2
  Demux/1 -> Mux/1
  Mux/1 -> For Even Sector/1("S1, S3, S1"), For Odd Sector/1("S1, S3, S5")
  Constant/1 -> Mod/2
  NOT/1 -> AND/2, AND1/2, AND2/2
  For Odd Sector/2(Gate 3 Pulse) -> AND4/1
  "S1, S3, S5, sector"/1 -> Demux/1
  AND3/1 -> OR/1

== system MATLAB Simulink Model/Space Vector PWM based VSI /Gating Pulse Generator/Gate Pulse Generator for 2721 Sequence ==
  "S1, S3, S5, sector" : Inport
  AND{,1..5} (6 alike) : Logic  IconShape=distinctive  AllPortsSameDT=off  OutDataTypeStr=boolean
  Constant : Constant  Value=2
  Data Type Conversion : DataTypeConversion
  Demux : Demux
  For Even Sector : Subsystem
  For Odd Sector : Subsystem
  Mod : Math  Operator=mod  SaturateOnIntegerOverflow=on
  Mux : Mux  Inputs=3
  NOT : Logic  Operator=NOT  IconShape=distinctive  AllPortsSameDT=off  OutDataTypeStr=boolean
  OR : Logic  Operator=OR  IconShape=distinctive  AllPortsSameDT=off  OutDataTypeStr=boolean
  OR1 : Logic  Operator=OR  IconShape=distinctive  AllPortsSameDT=off  OutDataTypeStr=boolean
  OR2 : Logic  Operator=OR  IconShape=distinctive  AllPortsSameDT=off  OutDataTypeStr=boolean
  Scope1 : Scope  NumInputPorts=4
  Gate 1 Pulse : Outport
  Gate 3 Pulse : Outport  Port=2
  Gate 5 Pulse : Outport  Port=3
  wires:
  For Odd Sector/3(Gate 5 Pulse) -> AND5/1
  For Odd Sector/1(Gate 1 Pulse) -> AND3/1
  For Even Sector/3(Gate 5 Pulse) -> AND2/1
  OR2/1 -> Scope1/3, Gate 5 Pulse/1
  For Even Sector/2(Gate 3 Pulse) -> AND1/1
  OR1/1 -> Scope1/2, Gate 3 Pulse/1
  Demux/3 -> Mux/3
  AND4/1 -> OR1/1
  OR/1 -> Scope1/1, Gate 1 Pulse/1
  AND5/1 -> OR2/1
  Demux/2 -> Mux/2
  For Odd Sector/2(Gate 3 Pulse) -> AND4/1
  AND1/1 -> OR1/2
  AND/1 -> OR/2
  Mod/1 -> Data Type Conversion/1
  Data Type Conversion/1 -> AND3/2, AND4/2, AND5/2, NOT/1
  AND2/1 -> OR2/2
  "S1, S3, S5, sector"/1 -> Demux/1
  AND3/1 -> OR/1
  Demux/4 -> Scope1/4, Mod/1
  Demux/1 -> Mux/1
  Mux/1 -> For Even Sector/1("S1, S3, S5"), For Odd Sector/1("S1, S3, S1")
  Constant/1 -> Mod/2
  NOT/1 -> AND/2, AND1/2, AND2/2
  For Even Sector/1(Gate 1 Pulse) -> AND/1

== system MATLAB Simulink Model/Space Vector PWM based VSI /Gating Pulse Generator/Gate Pulse Generator for 7212 Sequence ==
  "S1, S3, S5, sector" : Inport
  AND{,1..5} (6 alike) : Logic  IconShape=distinctive  AllPortsSameDT=off  OutDataTypeStr=boolean
  Constant : Constant  Value=2
  Data Type Conversion : DataTypeConversion
  Demux : Demux
  For Even Sector : Subsystem
  For Odd Sector : Subsystem
  Mod : Math  Operator=mod  SaturateOnIntegerOverflow=on
  Mux : Mux  Inputs=3
  NOT : Logic  Operator=NOT  IconShape=distinctive  AllPortsSameDT=off  OutDataTypeStr=boolean
  OR : Logic  Operator=OR  IconShape=distinctive  AllPortsSameDT=off  OutDataTypeStr=boolean
  OR1 : Logic  Operator=OR  IconShape=distinctive  AllPortsSameDT=off  OutDataTypeStr=boolean
  OR2 : Logic  Operator=OR  IconShape=distinctive  AllPortsSameDT=off  OutDataTypeStr=boolean
  Scope1 : Scope  NumInputPorts=4
  Gate 1 Pulse : Outport
  Gate 3 Pulse : Outport  Port=2
  Gate 5 Pulse : Outport  Port=3
  wires:
  For Odd Sector/3(Gate 5 Pulse) -> AND5/1
  For Odd Sector/1(Gate 1 Pulse) -> AND3/1
  For Even Sector/3(Gate 5 Pulse) -> AND2/1
  For Even Sector/2(Gate 3 Pulse) -> AND1/1
  OR2/1 -> Scope1/3, Gate 5 Pulse/1
  OR1/1 -> Scope1/2, Gate 3 Pulse/1
  Demux/3 -> Mux/3
  For Even Sector/1(Gate 1 Pulse) -> AND/1
  AND4/1 -> OR1/1
  OR/1 -> Scope1/1, Gate 1 Pulse/1
  AND5/1 -> OR2/1
  Demux/2 -> Mux/2
  AND1/1 -> OR1/2
  AND/1 -> OR/2
  Mod/1 -> Data Type Conversion/1
  Demux/4 -> Scope1/4, Mod/1
  Data Type Conversion/1 -> AND3/2, AND4/2, AND5/2, NOT/1
  AND2/1 -> OR2/2
  Demux/1 -> Mux/1
  Mux/1 -> For Even Sector/1("S1, S3, S1"), For Odd Sector/1("S1, S3, S5")
  Constant/1 -> Mod/2
  NOT/1 -> AND/2, AND1/2, AND2/2
  For Odd Sector/2(Gate 3 Pulse) -> AND4/1
  "S1, S3, S5, sector"/1 -> Demux/1
  AND3/1 -> OR/1

== system MATLAB Simulink Model/Space Vector PWM based VSI /Switching Times and Sector/Angle Calculation1 ==
  freq : Inport
  Delay : Delay  DelayLength=1  InitialCondition=0  UseCircularBuffer=on
  Gain1 : Gain  Gain=Tsys
  MATLAB Function : MATLAB Function  TreatAsAtomicUnit=on
  Scope : Scope
  Zero-Order Hold : ZeroOrderHold  SampleTime=Ts
  w : Gain  Gain=2*pi
  Angle : Outport
  tag scope: wt=global
  wires:
  freq/1 -> w/1, Scope/1
  Gain1/1 -> MATLAB Function/2(wTs)
  Zero-Order Hold/1 -> Angle/1
  Delay/1 -> MATLAB Function/1(wold)
  MATLAB Function/1(wnew) -> Delay/1, Zero-Order Hold/1, [wt]
  w/1 -> Gain1/1

== system MATLAB Simulink Model/Space Vector PWM based VSI 1/Gating Pulse Generator/Gate Pulse Generator for 0121 Sequence ==
  "S1, S3, S5, sector" : Inport
  AND{,1..5} (6 alike) : Logic  IconShape=distinctive  AllPortsSameDT=off  OutDataTypeStr=boolean
  Constant : Constant  Value=2
  Data Type Conversion : DataTypeConversion
  Demux : Demux
  For Even Sector : Subsystem
  For Odd Sector : Subsystem
  Mod : Math  Operator=mod  SaturateOnIntegerOverflow=on
  Mux : Mux  Inputs=3
  NOT : Logic  Operator=NOT  IconShape=distinctive  AllPortsSameDT=off  OutDataTypeStr=boolean
  OR : Logic  Operator=OR  IconShape=distinctive  AllPortsSameDT=off  OutDataTypeStr=boolean
  OR1 : Logic  Operator=OR  IconShape=distinctive  AllPortsSameDT=off  OutDataTypeStr=boolean
  OR2 : Logic  Operator=OR  IconShape=distinctive  AllPortsSameDT=off  OutDataTypeStr=boolean
  Scope1 : Scope  NumInputPorts=4
  Gate 1 Pulse : Outport
  Gate 3 Pulse : Outport  Port=2
  Gate 5 Pulse : Outport  Port=3
  wires:
  AND3/1 -> OR/1
  "S1, S3, S5, sector"/1 -> Demux/1
  Mod/1 -> Data Type Conversion/1
  NOT/1 -> AND2/2, AND1/2, AND/2
  Constant/1 -> Mod/2
  For Even Sector/2(Gate 3 Pulse) -> AND1/1
  Mux/1 -> For Odd Sector/1("S1, S3, S5"), For Even Sector/1("S1, S3, S5")
  Demux/1 -> Mux/1
  AND2/1 -> OR2/2
  Data Type Conversion/1 -> NOT/1, AND5/2, AND4/2, AND3/2
  For Even Sector/1(Gate 1 Pulse) -> AND/1
  For Odd Sector/2(Gate 3 Pulse) -> AND4/1
  For Even Sector/3(Gate 5 Pulse) -> AND2/1
  Demux/4 -> Mod/1, Scope1/4
  AND/1 -> OR/2
  AND1/1 -> OR1/2
  Demux/2 -> Mux/2
  AND5/1 -> OR2/1
  For Odd Sector/1(Gate 1 Pulse) -> AND3/1
  OR/1 -> Gate 1 Pulse/1, Scope1/1
  AND4/1 -> OR1/1
  Demux/3 -> Mux/3
  OR1/1 -> Gate 3 Pulse/1, Scope1/2
  OR2/1 -> Gate 5 Pulse/1, Scope1/3
  For Odd Sector/3(Gate 5 Pulse) -> AND5/1

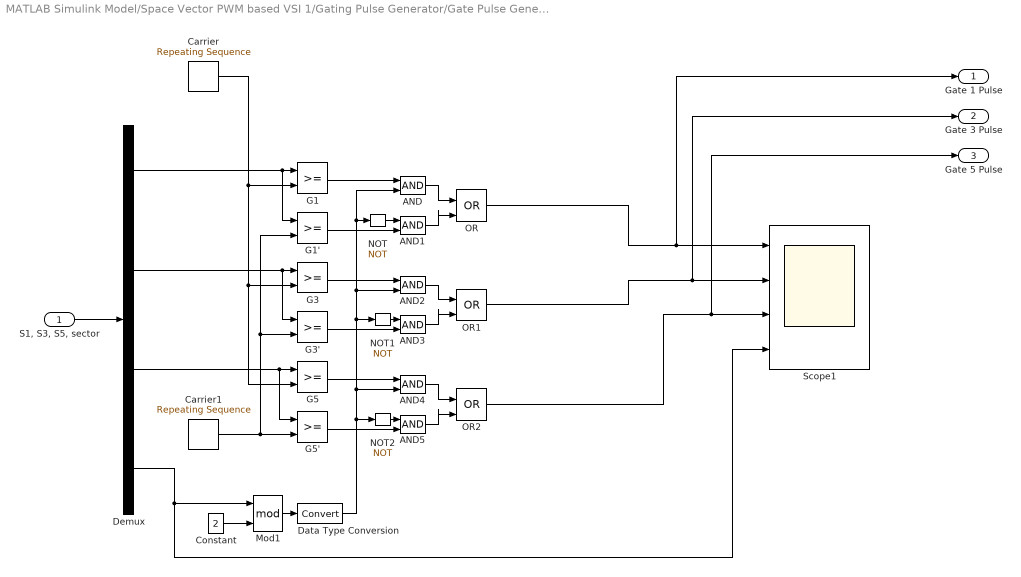
== system MATLAB Simulink Model/Space Vector PWM based VSI 1/Gating Pulse Generator/Gate Pulse Generator for 0127 Sequence ==
  "S1, S3, S5, sector" : Inport
  AND{,1..5} (6 alike) : Logic  IconShape=distinctive  AllPortsSameDT=off  OutDataTypeStr=boolean
  Carrier : simulink/Sources/Repeating Sequence  rep_seq_t=[0 Ts/2 Ts]  rep_seq_y=[Ts-(1e-16) 0 Ts-(1e-16)]
  Carrier1 : simulink/Sources/Repeating Sequence  rep_seq_t=[0 Ts/2 Ts]  rep_seq_y=[0 Ts-(1e-16) 0]
  Constant : Constant  Value=2
  Data Type Conversion : DataTypeConversion
  Demux : Demux
  G1 : RelationalOperator  OutDataTypeStr=boolean  RndMeth=Simplest
  G1' : RelationalOperator  OutDataTypeStr=boolean  RndMeth=Simplest
  G3 : RelationalOperator  OutDataTypeStr=boolean  RndMeth=Simplest
  G3' : RelationalOperator  OutDataTypeStr=boolean  RndMeth=Simplest
  G5 : RelationalOperator  OutDataTypeStr=boolean  RndMeth=Simplest
  G5' : RelationalOperator  OutDataTypeStr=boolean  RndMeth=Simplest
  Mod1 : Math  Operator=mod  SaturateOnIntegerOverflow=on
  NOT : Logic  Operator=NOT  IconShape=distinctive  AllPortsSameDT=off  OutDataTypeStr=boolean
  NOT1 : Logic  Operator=NOT  IconShape=distinctive  AllPortsSameDT=off  OutDataTypeStr=boolean
  NOT2 : Logic  Operator=NOT  IconShape=distinctive  AllPortsSameDT=off  OutDataTypeStr=boolean
  OR : Logic  Operator=OR  IconShape=distinctive  AllPortsSameDT=off  OutDataTypeStr=boolean
  OR1 : Logic  Operator=OR  IconShape=distinctive  AllPortsSameDT=off  OutDataTypeStr=boolean
  OR2 : Logic  Operator=OR  IconShape=distinctive  AllPortsSameDT=off  OutDataTypeStr=boolean
  Scope1 : Scope  NumInputPorts=4
  Gate 1 Pulse : Outport
  Gate 3 Pulse : Outport  Port=2
  Gate 5 Pulse : Outport  Port=3
  wires:
  Demux/3 -> G5/1, G5'/1
  Demux/2 -> G3/1, G3'/1
  Demux/4 -> Mod1/1, Scope1/4
  "S1, S3, S5, sector"/1 -> Demux/1
  AND2/1 -> OR1/1
  Carrier/1 -> G1/2, G3/2, G5/2
  G1/1 -> AND/1
  G1'/1 -> AND1/2
  Demux/1 -> G1/1, G1'/1
  Carrier1/1 -> G5'/2, G3'/2, G1'/2
  NOT1/1 -> AND3/1
  NOT2/1 -> AND5/1
  AND3/1 -> OR1/2
  Mod1/1 -> Data Type Conversion/1
  NOT/1 -> AND1/1
  OR1/1 -> Gate 3 Pulse/1, Scope1/2
  AND/1 -> OR/1
  AND4/1 -> OR2/1
  AND5/1 -> OR2/2
  G5/1 -> AND4/1
  G5'/1 -> AND5/2
  Data Type Conversion/1 -> AND/2, NOT/1, AND2/2, NOT1/1, AND4/2, NOT2/1
  AND1/1 -> OR/2
  Constant/1 -> Mod1/2
  OR/1 -> Scope1/1, Gate 1 Pulse/1
  G3'/1 -> AND3/2
  OR2/1 -> Scope1/3, Gate 5 Pulse/1
  G3/1 -> AND2/1

== system MATLAB Simulink Model/Space Vector PWM based VSI 1/Gating Pulse Generator/Gate Pulse Generator for 0127 Sequence 1 ==
  "S1, S3, S5, sector" : Inport
  AND{,1..5} (6 alike) : Logic  IconShape=distinctive  AllPortsSameDT=off  OutDataTypeStr=boolean
  Constant : Constant  Value=2
  Data Type Conversion : DataTypeConversion
  Demux : Demux
  For Even Sector : Subsystem
  For Odd Sector : Subsystem
  Mod : Math  Operator=mod  SaturateOnIntegerOverflow=on
  Mux : Mux  Inputs=3
  NOT : Logic  Operator=NOT  IconShape=distinctive  AllPortsSameDT=off  OutDataTypeStr=boolean
  OR : Logic  Operator=OR  IconShape=distinctive  AllPortsSameDT=off  OutDataTypeStr=boolean
  OR1 : Logic  Operator=OR  IconShape=distinctive  AllPortsSameDT=off  OutDataTypeStr=boolean
  OR2 : Logic  Operator=OR  IconShape=distinctive  AllPortsSameDT=off  OutDataTypeStr=boolean
  Scope1 : Scope  NumInputPorts=4
  Gate 1 Pulse : Outport
  Gate 3 Pulse : Outport  Port=2
  Gate 5 Pulse : Outport  Port=3
  wires:
  For Odd Sector/3(Gate 5 Pulse1) -> AND5/1
  For Odd Sector/2(Gate 3 Pulse1) -> AND4/1
  For Even Sector/3(Gate 5 Pulse) -> AND2/1
  For Even Sector/2(Gate 3 Pulse) -> AND1/1
  For Even Sector/1(Gate 1 Pulse) -> AND/1
  OR2/1 -> Gate 5 Pulse/1, Scope1/3
  OR/1 -> Gate 1 Pulse/1, Scope1/1
  OR1/1 -> Gate 3 Pulse/1, Scope1/2
  AND2/1 -> OR2/2
  AND5/1 -> OR2/1
  AND1/1 -> OR1/2
  AND4/1 -> OR1/1
  AND/1 -> OR/2
  AND3/1 -> OR/1
  Data Type Conversion/1 -> NOT/1, AND5/2, AND4/2, AND3/2
  For Odd Sector/1(Gate 1 Pulse1) -> AND3/1
  NOT/1 -> AND2/2, AND1/2, AND/2
  Mod/1 -> Data Type Conversion/1
  Constant/1 -> Mod/2
  Demux/4 -> Mod/1, Scope1/4
  Mux/1 -> For Odd Sector/1("S1, S3, S1"), For Even Sector/1("S1, S3, S5")
  Demux/3 -> Mux/3
  Demux/2 -> Mux/2
  Demux/1 -> Mux/1
  "S1, S3, S5, sector"/1 -> Demux/1

== system MATLAB Simulink Model/Space Vector PWM based VSI 1/Gating Pulse Generator/Gate Pulse Generator for 1012 Sequence ==
  "S1, S3, S5, sector" : Inport
  AND{,1..5} (6 alike) : Logic  IconShape=distinctive  AllPortsSameDT=off  OutDataTypeStr=boolean
  Constant : Constant  Value=2
  Data Type Conversion : DataTypeConversion
  Demux : Demux
  For Even Sector : Subsystem
  For Odd Sector : Subsystem
  Mod : Math  Operator=mod  SaturateOnIntegerOverflow=on
  Mux : Mux  Inputs=3
  NOT : Logic  Operator=NOT  IconShape=distinctive  AllPortsSameDT=off  OutDataTypeStr=boolean
  OR : Logic  Operator=OR  IconShape=distinctive  AllPortsSameDT=off  OutDataTypeStr=boolean
  OR1 : Logic  Operator=OR  IconShape=distinctive  AllPortsSameDT=off  OutDataTypeStr=boolean
  OR2 : Logic  Operator=OR  IconShape=distinctive  AllPortsSameDT=off  OutDataTypeStr=boolean
  Scope1 : Scope  NumInputPorts=4
  Gate 1 Pulse : Outport
  Gate 3 Pulse : Outport  Port=2
  Gate 5 Pulse : Outport  Port=3
  wires:
  AND3/1 -> OR/1
  "S1, S3, S5, sector"/1 -> Demux/1
  For Odd Sector/2(Gate 3 Pulse) -> AND4/1
  NOT/1 -> AND2/2, AND1/2, AND/2
  Constant/1 -> Mod/2
  Mux/1 -> For Odd Sector/1("S1, S3, S5"), For Even Sector/1("S1, S3, S1")
  Demux/1 -> Mux/1
  AND2/1 -> OR2/2
  Data Type Conversion/1 -> NOT/1, AND5/2, AND4/2, AND3/2
  Demux/4 -> Mod/1, Scope1/4
  Mod/1 -> Data Type Conversion/1
  AND/1 -> OR/2
  AND1/1 -> OR1/2
  Demux/2 -> Mux/2
  AND5/1 -> OR2/1
  OR/1 -> Gate 1 Pulse/1, Scope1/1
  AND4/1 -> OR1/1
  For Even Sector/1(Gate 1 Pulse) -> AND/1
  Demux/3 -> Mux/3
  OR1/1 -> Gate 3 Pulse/1, Scope1/2
  OR2/1 -> Gate 5 Pulse/1, Scope1/3
  For Even Sector/2(Gate 3 Pulse) -> AND1/1
  For Even Sector/3(Gate 5 Pulse) -> AND2/1
  For Odd Sector/1(Gate 1 Pulse) -> AND3/1
  For Odd Sector/3(Gate 5 Pulse) -> AND5/1
